simulink model "ScriptDemo"  (R2022b)
settings: configuration reference "TmVcThermal_Configuration_sub" (kept outside this file)
undefined symbols (not defined in the file): aaaa, bbbb, cTmComprCtrl_D_u8HvacFlowTable_db, cTmComprCtrl_D_u8HvacFlowTable_sw, cTmComprCtrl_n_i16ChillCmpIMax, cTmComprCtrl_n_i16ChillCmpIMin, cTmComprCtrl_n_i16ChillCmpIMin666, cTmComprCtrl_n_i16ChillCmpPMax, cTmComprCtrl_n_i16ChillCmpPMin, cTmComprCtrl_n_i16CmpChillCoolRpmKiMax, cTmComprCtrl_n_i16CmpChillCoolRpmKiMin, cTmComprCtrl_n_i16CmpChillCoolRpmKpMax, cTmComprCtrl_n_i16CmpChillCoolRpmKpMin, cTmComprCtrl_n_i16CmpCoolRpmKiMax, cTmComprCtrl_n_i16CmpCoolRpmKiMin, cTmComprCtrl_n_i16CmpCoolRpmKpMax, cTmComprCtrl_n_i16CmpCoolRpmKpMin, cTmComprCtrl_n_i16SM4CmpHeatKiMax, cTmComprCtrl_n_i16SM4CmpHeatKiMin, cTmComprCtrl_n_i16SM4CmpHeatKpMax, cTmComprCtrl_n_i16SM4CmpHeatKpMin, cTmComprCtrl_n_i16SM5CmpHeatKiMax, cTmComprCtrl_n_i16SM5CmpHeatKiMin, cTmComprCtrl_n_i16SM5CmpHeatKpMax, cTmComprCtrl_n_i16SM5CmpHeatKpMin, cTmComprCtrl_n_i16SM6CmpHeatKiMax, cTmComprCtrl_n_i16SM6CmpHeatKiMin, cTmComprCtrl_n_i16SM6CmpHeatKpMax, cTmComprCtrl_n_i16SM6CmpHeatKpMin, cTmComprCtrl_n_u16CmpMaxSpdFanFltLimt, cTmComprCtrl_n_u16CmpMaxSpdLoSidePFltLimt, cTmComprCtrl_n_u16CmpMaxSpdSensorFltLimt, cTmComprCtrl_n_u16CompMinRpm, cTmComprCtrl_n_u16CompRpmIncThres, cTmComprCtrl_t_u16BattCooltFFPeriod, cTmComprCtrl_t_u16BattCooltPIPeriod, cTmComprCtrl_t_u16CmpCoolFFPeriod, cTmComprCtrl_t_u16CmpCoolPIPeriod, cTmComprCtrl_t_u16CoolCmpChillFFPeriod, cTmComprCtrl_t_u16CoolCmpChillPIPeriod, cTmComprCtrl_t_u16SM4CmpHeatFFPeriod, cTmComprCtrl_t_u16SM4CmpHeatPIPeriod, cTmComprCtrl_t_u16SM5CmpHeatFFPeriod, cTmComprCtrl_t_u16SM5CmpHeatPIPeriod, cTmComprCtrl_t_u16SM6CmpHeatFFPeriod, cTmComprCtrl_t_u16SM6CmpHeatPIPeriod, cTmComprCtrl_Te_EvapClearInteg, cTmComprCtrl_Te_i16HpReqTempSaturoffset, cTmComprCtrl_Te_i16SatLpReplaceDiff, cTmComprCtrl_Te_i16SM3BatDiffStartEvapDecOffset, cTmComprCtrl_Te_i16SM3EvapLo, cTmComprCtrl_Te_i16SM3TBatDiffEntEvapDecOffset, cTmComprCtrl_Te_i16SM3TBatDiffEntEvapDecOffsetQuit, cTmComprCtrl_Te_s32ErrCmpChillPIContinueCoolH, cTmComprCtrl_Te_s32ErrCmpChillPIContinueCoolL, cTmComprCtrl_Te_s32ErrCmpPIContinueChillH, cTmComprCtrl_Te_s32ErrCmpPIContinueChillL, cTmComprCtrl_Te_s32ErrCmpPIContinueCoolH, cTmComprCtrl_Te_s32ErrCmpPIContinueCoolL, cTmComprCtrl_Te_s32ErrCmpPIContinueHeatH ... (+398)
libraries: simulink x782, PCMULib x640, simulink_need_slupdate x4
(part 27 of 41)

== system ScriptDemo/Create/createMerge/Before/SM2SM22/ID26239_SM2Error/NegAndPosCheck 1 ==
  SetPoint : Inport
  Acture : Inport  Port=2
  Compare To Constant : simulink/Logic and Bit Operations/Compare To Constant  relop=>=  const=0  OutDataTypeStr=boolean
  Data Type Conversion : DataTypeConversion  SaturateOnIntegerOverflow=off  RndMeth=Floor
  Data Type Conversion1 : DataTypeConversion  SaturateOnIntegerOverflow=off  RndMeth=Floor
  Data Type Conversion2 : DataTypeConversion  SaturateOnIntegerOverflow=off  RndMeth=Floor
  Sum : Sum  Inputs=|-+  OutDataTypeStr=Inherit: Same as first input
  Dvt : Outport  VectorParamsAs1DForOutWhenUnconnected=off
  Dvt_PosFlag : Outport  Port=2  VectorParamsAs1DForOutWhenUnconnected=off
  wires:
  Data Type Conversion2/1 -> Dvt/1, Compare To Constant/1
  Data Type Conversion1/1 -> Sum/2
  Data Type Conversion/1 -> Sum/1
  Compare To Constant/1 -> Dvt_PosFlag/1
  Sum/1 -> Data Type Conversion2/1
  Acture/1 -> Data Type Conversion1/1
  SetPoint/1 -> Data Type Conversion/1

== system ScriptDemo/Create/createMerge/Before/SM2SM22/ID26267_SM2FF/Flow2RpmOsa ==
  md_u8Blw : Inport
  breakpoint1 : Inport  Port=2
  breakpoint2 : Inport  Port=3
  2-D Lookup Table5 : Lookup_n-D  BreakpointsForDimension1=FFBlw1_Y  BreakpointsForDimension2=FFBlw1_X  BreakpointsForDimension1DataTypeStr=Inherit: Inherit from 'Breakpoint data'  BreakpointsForDimension2DataTypeStr=Inherit: Inherit from 'Breakpoint data'  Table=FFBlw1  TableDataTypeStr=Inherit: Inherit from 'Table data'  ExtrapMethod=Clip  InternalRulePriority=Speed  OutDataTypeStr=Inherit: Inherit from 'Table data'  RndMeth=Simplest
      settings: InputPortMap=u0,u1
  2-D Lookup Table6 : Lookup_n-D  BreakpointsForDimension1=FFBlw3_Y  BreakpointsForDimension2=FFBlw3_X  BreakpointsForDimension1DataTypeStr=Inherit: Inherit from 'Breakpoint data'  BreakpointsForDimension2DataTypeStr=Inherit: Inherit from 'Breakpoint data'  Table=FFBlw3  TableDataTypeStr=Inherit: Inherit from 'Table data'  ExtrapMethod=Clip  InternalRulePriority=Speed  OutDataTypeStr=Inherit: Inherit from 'Table data'  RndMeth=Simplest
      settings: InputPortMap=u0,u1
  2-D Lookup Table7 : Lookup_n-D  BreakpointsForDimension1=FFBlw5_Y  BreakpointsForDimension2=FFBlw5_X  BreakpointsForDimension1DataTypeStr=Inherit: Inherit from 'Breakpoint data'  BreakpointsForDimension2DataTypeStr=Inherit: Inherit from 'Breakpoint data'  Table=FFBlw5  TableDataTypeStr=Inherit: Inherit from 'Table data'  ExtrapMethod=Clip  InternalRulePriority=Speed  OutDataTypeStr=Inherit: Inherit from 'Table data'  RndMeth=Simplest
      settings: InputPortMap=u0,u1
  2-D Lookup Table8 : Lookup_n-D  BreakpointsForDimension1=FFBlw7_Y  BreakpointsForDimension2=FFBlw7_X  BreakpointsForDimension1DataTypeStr=Inherit: Inherit from 'Breakpoint data'  BreakpointsForDimension2DataTypeStr=Inherit: Inherit from 'Breakpoint data'  Table=FFBlw7  TableDataTypeStr=Inherit: Inherit from 'Table data'  ExtrapMethod=Clip  InternalRulePriority=Speed  OutDataTypeStr=Inherit: Inherit from 'Table data'  RndMeth=Simplest
      settings: InputPortMap=u0,u1
  2-D Lookup Table9 : Lookup_n-D  BreakpointsForDimension1=FFBlw9_Y  BreakpointsForDimension2=FFBlw9_X  BreakpointsForDimension1DataTypeStr=Inherit: Inherit from 'Breakpoint data'  BreakpointsForDimension2DataTypeStr=Inherit: Inherit from 'Breakpoint data'  Table=FFBlw9  TableDataTypeStr=Inherit: Inherit from 'Table data'  ExtrapMethod=Clip  InternalRulePriority=Speed  OutDataTypeStr=Inherit: Inherit from 'Table data'  RndMeth=Simplest
      settings: InputPortMap=u0,u1
  Add{2..6} (5 alike) : Sum  Inputs=+-  OutDataTypeStr=int16
  Add7 : Sum  Inputs=+++++
  Constant{,1..4} (5 alike) : Constant  Value=0.1  OutDataTypeStr=single
  Constant5 : Constant  Value=10  OutDataTypeStr=int16
  Constant6 : Constant  Value=20  OutDataTypeStr=int16
  Constant7 : Constant  Value=30  OutDataTypeStr=int16
  Constant8 : Constant  Value=40  OutDataTypeStr=int16
  Constant9 : Constant  Value=50  OutDataTypeStr=int16
  Data Type Conversion : DataTypeConversion  OutDataTypeStr=uint16  SaturateOnIntegerOverflow=off  RndMeth=Floor
  Data Type Conversion1 : DataTypeConversion  OutDataTypeStr=int16  SaturateOnIntegerOverflow=off  RndMeth=Floor
  Product{,1..9} (10 alike) : Product  OutDataTypeStr=single
  Subsystem1 : Subsystem
  Subsystem2 : Subsystem
  Subsystem3 : Subsystem
  Subsystem4 : Subsystem
  Subsystem5 : Subsystem
  XCP : Subsystem
  Flow2Rpm : Outport
  wires:
  Subsystem1/1(Out1) -> Product/2
  Product2/1 -> Product7/2
  [breakpoint2] -> 2-D Lookup Table5/2
  Product4/1 -> Product9/2
  Product9/1 -> Add7/5
  [breakpoint1] -> 2-D Lookup Table7/1
  Constant9/1 -> Add6/1
  [breakpoint1] -> 2-D Lookup Table9/1
  [breakpoint1] -> 2-D Lookup Table5/1
  [breakpoint1] -> 2-D Lookup Table6/1
  Product5/1 -> Add7/1
  2-D Lookup Table7/1 -> Product2/1
  Data Type Conversion1/1 -> Add4/2, Add6/2, Add5/2, Add3/2, Add2/2
  [breakpoint2] -> 2-D Lookup Table8/2
  Product/1 -> Product5/2
  Subsystem5/1(Out1) -> Product4/2
  [breakpoint2] -> 2-D Lookup Table7/2
  Subsystem2/1(Out1) -> Product1/2
  Constant8/1 -> Add5/1
  Product8/1 -> Add7/4
  Constant7/1 -> Add4/1
  Add4/1 -> Subsystem3/1(In1)
  Subsystem3/1(Out1) -> Product2/2
  Subsystem4/1(Out1) -> Product3/2
  Product1/1 -> Product6/2
  Add2/1 -> Subsystem1/1(In1)
  [breakpoint1] -> 2-D Lookup Table8/1
  [breakpoint2] -> 2-D Lookup Table6/2
  2-D Lookup Table5/1 -> Product/1
  Constant5/1 -> Add2/1
  2-D Lookup Table8/1 -> Product3/1
  Constant6/1 -> Add3/1
  Add6/1 -> Subsystem5/1(In1)
  Add5/1 -> Subsystem4/1(In1)
  Product3/1 -> Product8/2
  [breakpoint2] -> 2-D Lookup Table9/2
  Add3/1 -> Subsystem2/1(In1)
  Add7/1 -> Data Type Conversion/1
  2-D Lookup Table6/1 -> Product1/1
  Product7/1 -> Add7/3
  2-D Lookup Table9/1 -> Product4/1
  Product6/1 -> Add7/2
  breakpoint1/1 -> [breakpoint1]
  breakpoint2/1 -> [breakpoint2]
  XCP/1(Out1) -> Data Type Conversion1/1
  Constant/1 -> Product5/1
  Constant1/1 -> Product6/1
  Constant2/1 -> Product7/1
  Constant3/1 -> Product8/1
  Constant4/1 -> Product9/1
  md_u8Blw/1 -> XCP/1(md_u8Blw)
  Data Type Conversion/1 -> Flow2Rpm/1

== system ScriptDemo/Create/createMerge/Before/SM2SM22/ID26267_SM2FF/Flow2RpmOsa1 ==
  md_u8Blw : Inport
  breakpoint1 : Inport  Port=2
  breakpoint2 : Inport  Port=3
  2-D Lookup Table5 : Lookup_n-D  BreakpointsForDimension1=FFBlw1_Y  BreakpointsForDimension2=FFBlw1_X  BreakpointsForDimension1DataTypeStr=Inherit: Inherit from 'Breakpoint data'  BreakpointsForDimension2DataTypeStr=Inherit: Inherit from 'Breakpoint data'  Table=FFBlw1  TableDataTypeStr=Inherit: Inherit from 'Table data'  ExtrapMethod=Clip  InternalRulePriority=Speed  OutDataTypeStr=Inherit: Inherit from 'Table data'  RndMeth=Simplest
      settings: InputPortMap=u0,u1
  2-D Lookup Table6 : Lookup_n-D  BreakpointsForDimension1=FFBlw3_Y  BreakpointsForDimension2=FFBlw3_X  BreakpointsForDimension1DataTypeStr=Inherit: Inherit from 'Breakpoint data'  BreakpointsForDimension2DataTypeStr=Inherit: Inherit from 'Breakpoint data'  Table=FFBlw3  TableDataTypeStr=Inherit: Inherit from 'Table data'  ExtrapMethod=Clip  InternalRulePriority=Speed  OutDataTypeStr=Inherit: Inherit from 'Table data'  RndMeth=Simplest
      settings: InputPortMap=u0,u1
  2-D Lookup Table7 : Lookup_n-D  BreakpointsForDimension1=FFBlw5_Y  BreakpointsForDimension2=FFBlw5_X  BreakpointsForDimension1DataTypeStr=Inherit: Inherit from 'Breakpoint data'  BreakpointsForDimension2DataTypeStr=Inherit: Inherit from 'Breakpoint data'  Table=FFBlw5  TableDataTypeStr=Inherit: Inherit from 'Table data'  ExtrapMethod=Clip  InternalRulePriority=Speed  OutDataTypeStr=Inherit: Inherit from 'Table data'  RndMeth=Simplest
      settings: InputPortMap=u0,u1
  2-D Lookup Table8 : Lookup_n-D  BreakpointsForDimension1=FFBlw7_Y  BreakpointsForDimension2=FFBlw7_X  BreakpointsForDimension1DataTypeStr=Inherit: Inherit from 'Breakpoint data'  BreakpointsForDimension2DataTypeStr=Inherit: Inherit from 'Breakpoint data'  Table=FFBlw7  TableDataTypeStr=Inherit: Inherit from 'Table data'  ExtrapMethod=Clip  InternalRulePriority=Speed  OutDataTypeStr=Inherit: Inherit from 'Table data'  RndMeth=Simplest
      settings: InputPortMap=u0,u1
  2-D Lookup Table9 : Lookup_n-D  BreakpointsForDimension1=FFBlw9_Y  BreakpointsForDimension2=FFBlw9_X  BreakpointsForDimension1DataTypeStr=Inherit: Inherit from 'Breakpoint data'  BreakpointsForDimension2DataTypeStr=Inherit: Inherit from 'Breakpoint data'  Table=FFBlw9  TableDataTypeStr=Inherit: Inherit from 'Table data'  ExtrapMethod=Clip  InternalRulePriority=Speed  OutDataTypeStr=Inherit: Inherit from 'Table data'  RndMeth=Simplest
      settings: InputPortMap=u0,u1
  Add{2..6} (5 alike) : Sum  Inputs=+-  OutDataTypeStr=int16
  Add7 : Sum  Inputs=+++++
  Constant{,1..4} (5 alike) : Constant  Value=0.1  OutDataTypeStr=single
  Constant5 : Constant  Value=10  OutDataTypeStr=int16
  Constant6 : Constant  Value=20  OutDataTypeStr=int16
  Constant7 : Constant  Value=30  OutDataTypeStr=int16
  Constant8 : Constant  Value=40  OutDataTypeStr=int16
  Constant9 : Constant  Value=50  OutDataTypeStr=int16
  Data Type Conversion : DataTypeConversion  OutDataTypeStr=uint16  SaturateOnIntegerOverflow=off  RndMeth=Floor
  Data Type Conversion1 : DataTypeConversion  OutDataTypeStr=int16  SaturateOnIntegerOverflow=off  RndMeth=Floor
  Product{,1..9} (10 alike) : Product  OutDataTypeStr=single
  Subsystem1 : Subsystem
  Subsystem2 : Subsystem
  Subsystem3 : Subsystem
  Subsystem4 : Subsystem
  Subsystem5 : Subsystem
  XCP : Subsystem
  Flow2Rpm : Outport
  wires:
  Subsystem1/1(Out1) -> Product/2
  Product2/1 -> Product7/2
  [breakpoint2] -> 2-D Lookup Table5/2
  Product4/1 -> Product9/2
  Product9/1 -> Add7/5
  [breakpoint1] -> 2-D Lookup Table7/1
  Constant9/1 -> Add6/1
  [breakpoint1] -> 2-D Lookup Table9/1
  [breakpoint1] -> 2-D Lookup Table5/1
  [breakpoint1] -> 2-D Lookup Table6/1
  Product5/1 -> Add7/1
  2-D Lookup Table7/1 -> Product2/1
  Data Type Conversion1/1 -> Add4/2, Add6/2, Add5/2, Add3/2, Add2/2
  [breakpoint2] -> 2-D Lookup Table8/2
  Product/1 -> Product5/2
  Subsystem5/1(Out1) -> Product4/2
  [breakpoint2] -> 2-D Lookup Table7/2
  Subsystem2/1(Out1) -> Product1/2
  Constant8/1 -> Add5/1
  Product8/1 -> Add7/4
  Constant7/1 -> Add4/1
  Add4/1 -> Subsystem3/1(In1)
  Subsystem3/1(Out1) -> Product2/2
  Subsystem4/1(Out1) -> Product3/2
  Product1/1 -> Product6/2
  Add2/1 -> Subsystem1/1(In1)
  [breakpoint1] -> 2-D Lookup Table8/1
  [breakpoint2] -> 2-D Lookup Table6/2
  2-D Lookup Table5/1 -> Product/1
  Constant5/1 -> Add2/1
  2-D Lookup Table8/1 -> Product3/1
  Constant6/1 -> Add3/1
  Add6/1 -> Subsystem5/1(In1)
  Add5/1 -> Subsystem4/1(In1)
  Product3/1 -> Product8/2
  [breakpoint2] -> 2-D Lookup Table9/2
  Add3/1 -> Subsystem2/1(In1)
  Add7/1 -> Data Type Conversion/1
  2-D Lookup Table6/1 -> Product1/1
  Product7/1 -> Add7/3
  2-D Lookup Table9/1 -> Product4/1
  Product6/1 -> Add7/2
  breakpoint1/1 -> [breakpoint1]
  breakpoint2/1 -> [breakpoint2]
  XCP/1(Out1) -> Data Type Conversion1/1
  Constant/1 -> Product5/1
  Constant1/1 -> Product6/1
  Constant2/1 -> Product7/1
  Constant3/1 -> Product8/1
  Constant4/1 -> Product9/1
  md_u8Blw/1 -> XCP/1(md_u8Blw)
  Data Type Conversion/1 -> Flow2Rpm/1

== system ScriptDemo/Create/createMerge/Before/SM2SM22/ID26267_SM2FF/Flow2RpmRec ==
  md_u8Blw : Inport
  breakpoint1 : Inport  Port=2
  breakpoint2 : Inport  Port=3
  2-D Lookup Table5 : Lookup_n-D  BreakpointsForDimension1=FFBlw1_Y  BreakpointsForDimension2=FFBlw1_X  BreakpointsForDimension1DataTypeStr=Inherit: Inherit from 'Breakpoint data'  BreakpointsForDimension2DataTypeStr=Inherit: Inherit from 'Breakpoint data'  Table=FFBlw1  TableDataTypeStr=Inherit: Inherit from 'Table data'  ExtrapMethod=Clip  InternalRulePriority=Speed  OutDataTypeStr=Inherit: Inherit from 'Table data'  RndMeth=Simplest
      settings: InputPortMap=u0,u1
  2-D Lookup Table6 : Lookup_n-D  BreakpointsForDimension1=FFBlw3_Y  BreakpointsForDimension2=FFBlw3_X  BreakpointsForDimension1DataTypeStr=Inherit: Inherit from 'Breakpoint data'  BreakpointsForDimension2DataTypeStr=Inherit: Inherit from 'Breakpoint data'  Table=FFBlw3  TableDataTypeStr=Inherit: Inherit from 'Table data'  ExtrapMethod=Clip  InternalRulePriority=Speed  OutDataTypeStr=Inherit: Inherit from 'Table data'  RndMeth=Simplest
      settings: InputPortMap=u0,u1
  2-D Lookup Table7 : Lookup_n-D  BreakpointsForDimension1=FFBlw5_Y  BreakpointsForDimension2=FFBlw5_X  BreakpointsForDimension1DataTypeStr=Inherit: Inherit from 'Breakpoint data'  BreakpointsForDimension2DataTypeStr=Inherit: Inherit from 'Breakpoint data'  Table=FFBlw5  TableDataTypeStr=Inherit: Inherit from 'Table data'  ExtrapMethod=Clip  InternalRulePriority=Speed  OutDataTypeStr=Inherit: Inherit from 'Table data'  RndMeth=Simplest
      settings: InputPortMap=u0,u1
  2-D Lookup Table8 : Lookup_n-D  BreakpointsForDimension1=FFBlw7_Y  BreakpointsForDimension2=FFBlw7_X  BreakpointsForDimension1DataTypeStr=Inherit: Inherit from 'Breakpoint data'  BreakpointsForDimension2DataTypeStr=Inherit: Inherit from 'Breakpoint data'  Table=FFBlw7  TableDataTypeStr=Inherit: Inherit from 'Table data'  ExtrapMethod=Clip  InternalRulePriority=Speed  OutDataTypeStr=Inherit: Inherit from 'Table data'  RndMeth=Simplest
      settings: InputPortMap=u0,u1
  2-D Lookup Table9 : Lookup_n-D  BreakpointsForDimension1=FFBlw9_Y  BreakpointsForDimension2=FFBlw9_X  BreakpointsForDimension1DataTypeStr=Inherit: Inherit from 'Breakpoint data'  BreakpointsForDimension2DataTypeStr=Inherit: Inherit from 'Breakpoint data'  Table=FFBlw9  TableDataTypeStr=Inherit: Inherit from 'Table data'  ExtrapMethod=Clip  InternalRulePriority=Speed  OutDataTypeStr=Inherit: Inherit from 'Table data'  RndMeth=Simplest
      settings: InputPortMap=u0,u1
  Add{2..6} (5 alike) : Sum  Inputs=+-  OutDataTypeStr=int16
  Add7 : Sum  Inputs=+++++
  Constant{,1..4} (5 alike) : Constant  Value=0.1  OutDataTypeStr=single
  Constant5 : Constant  Value=10  OutDataTypeStr=int16
  Constant6 : Constant  Value=20  OutDataTypeStr=int16
  Constant7 : Constant  Value=30  OutDataTypeStr=int16
  Constant8 : Constant  Value=40  OutDataTypeStr=int16
  Constant9 : Constant  Value=50  OutDataTypeStr=int16
  Data Type Conversion : DataTypeConversion  OutDataTypeStr=uint16  SaturateOnIntegerOverflow=off  RndMeth=Floor
  Data Type Conversion1 : DataTypeConversion  OutDataTypeStr=int16  SaturateOnIntegerOverflow=off  RndMeth=Floor
  Product{,1..9} (10 alike) : Product  OutDataTypeStr=single
  Subsystem1 : Subsystem
  Subsystem2 : Subsystem
  Subsystem3 : Subsystem
  Subsystem4 : Subsystem
  Subsystem5 : Subsystem
  XCP : Subsystem
  Flow2Rpm : Outport
  wires:
  Subsystem1/1(Out1) -> Product/2
  Product2/1 -> Product7/2
  [breakpoint2] -> 2-D Lookup Table5/2
  Product4/1 -> Product9/2
  Product9/1 -> Add7/5
  [breakpoint1] -> 2-D Lookup Table7/1
  Constant9/1 -> Add6/1
  [breakpoint1] -> 2-D Lookup Table9/1
  [breakpoint1] -> 2-D Lookup Table5/1
  [breakpoint1] -> 2-D Lookup Table6/1
  Product5/1 -> Add7/1
  2-D Lookup Table7/1 -> Product2/1
  Data Type Conversion1/1 -> Add4/2, Add6/2, Add5/2, Add3/2, Add2/2
  [breakpoint2] -> 2-D Lookup Table8/2
  Product/1 -> Product5/2
  Subsystem5/1(Out1) -> Product4/2
  [breakpoint2] -> 2-D Lookup Table7/2
  Subsystem2/1(Out1) -> Product1/2
  Constant8/1 -> Add5/1
  Product8/1 -> Add7/4
  Constant7/1 -> Add4/1
  Add4/1 -> Subsystem3/1(In1)
  Subsystem3/1(Out1) -> Product2/2
  Subsystem4/1(Out1) -> Product3/2
  Product1/1 -> Product6/2
  Add2/1 -> Subsystem1/1(In1)
  [breakpoint1] -> 2-D Lookup Table8/1
  [breakpoint2] -> 2-D Lookup Table6/2
  2-D Lookup Table5/1 -> Product/1
  Constant5/1 -> Add2/1
  2-D Lookup Table8/1 -> Product3/1
  Constant6/1 -> Add3/1
  Add6/1 -> Subsystem5/1(In1)
  Add5/1 -> Subsystem4/1(In1)
  Product3/1 -> Product8/2
  [breakpoint2] -> 2-D Lookup Table9/2
  Add3/1 -> Subsystem2/1(In1)
  Add7/1 -> Data Type Conversion/1
  2-D Lookup Table6/1 -> Product1/1
  Product7/1 -> Add7/3
  2-D Lookup Table9/1 -> Product4/1
  Product6/1 -> Add7/2
  breakpoint1/1 -> [breakpoint1]
  breakpoint2/1 -> [breakpoint2]
  XCP/1(Out1) -> Data Type Conversion1/1
  Constant/1 -> Product5/1
  Constant1/1 -> Product6/1
  Constant2/1 -> Product7/1
  Constant3/1 -> Product8/1
  Constant4/1 -> Product9/1
  md_u8Blw/1 -> XCP/1(md_u8Blw)
  Data Type Conversion/1 -> Flow2Rpm/1

== system ScriptDemo/Create/createMerge/Before/SM2SM22/ID26267_SM2FF/Flow2RpmRec1 ==
  md_u8Blw : Inport
  breakpoint1 : Inport  Port=2
  breakpoint2 : Inport  Port=3
  2-D Lookup Table5 : Lookup_n-D  BreakpointsForDimension1=FFBlw1_Y  BreakpointsForDimension2=FFBlw1_X  BreakpointsForDimension1DataTypeStr=Inherit: Inherit from 'Breakpoint data'  BreakpointsForDimension2DataTypeStr=Inherit: Inherit from 'Breakpoint data'  Table=FFBlw1  TableDataTypeStr=Inherit: Inherit from 'Table data'  ExtrapMethod=Clip  InternalRulePriority=Speed  OutDataTypeStr=Inherit: Inherit from 'Table data'  RndMeth=Simplest
      settings: InputPortMap=u0,u1
  2-D Lookup Table6 : Lookup_n-D  BreakpointsForDimension1=FFBlw3_Y  BreakpointsForDimension2=FFBlw3_X  BreakpointsForDimension1DataTypeStr=Inherit: Inherit from 'Breakpoint data'  BreakpointsForDimension2DataTypeStr=Inherit: Inherit from 'Breakpoint data'  Table=FFBlw3  TableDataTypeStr=Inherit: Inherit from 'Table data'  ExtrapMethod=Clip  InternalRulePriority=Speed  OutDataTypeStr=Inherit: Inherit from 'Table data'  RndMeth=Simplest
      settings: InputPortMap=u0,u1
  2-D Lookup Table7 : Lookup_n-D  BreakpointsForDimension1=FFBlw5_Y  BreakpointsForDimension2=FFBlw5_X  BreakpointsForDimension1DataTypeStr=Inherit: Inherit from 'Breakpoint data'  BreakpointsForDimension2DataTypeStr=Inherit: Inherit from 'Breakpoint data'  Table=FFBlw5  TableDataTypeStr=Inherit: Inherit from 'Table data'  ExtrapMethod=Clip  InternalRulePriority=Speed  OutDataTypeStr=Inherit: Inherit from 'Table data'  RndMeth=Simplest
      settings: InputPortMap=u0,u1
  2-D Lookup Table8 : Lookup_n-D  BreakpointsForDimension1=FFBlw7_Y  BreakpointsForDimension2=FFBlw7_X  BreakpointsForDimension1DataTypeStr=Inherit: Inherit from 'Breakpoint data'  BreakpointsForDimension2DataTypeStr=Inherit: Inherit from 'Breakpoint data'  Table=FFBlw7  TableDataTypeStr=Inherit: Inherit from 'Table data'  ExtrapMethod=Clip  InternalRulePriority=Speed  OutDataTypeStr=Inherit: Inherit from 'Table data'  RndMeth=Simplest
      settings: InputPortMap=u0,u1
  2-D Lookup Table9 : Lookup_n-D  BreakpointsForDimension1=FFBlw9_Y  BreakpointsForDimension2=FFBlw9_X  BreakpointsForDimension1DataTypeStr=Inherit: Inherit from 'Breakpoint data'  BreakpointsForDimension2DataTypeStr=Inherit: Inherit from 'Breakpoint data'  Table=FFBlw9  TableDataTypeStr=Inherit: Inherit from 'Table data'  ExtrapMethod=Clip  InternalRulePriority=Speed  OutDataTypeStr=Inherit: Inherit from 'Table data'  RndMeth=Simplest
      settings: InputPortMap=u0,u1
  Add{2..6} (5 alike) : Sum  Inputs=+-  OutDataTypeStr=int16
  Add7 : Sum  Inputs=+++++
  Constant{,1..4} (5 alike) : Constant  Value=0.1  OutDataTypeStr=single
  Constant5 : Constant  Value=10  OutDataTypeStr=int16
  Constant6 : Constant  Value=20  OutDataTypeStr=int16
  Constant7 : Constant  Value=30  OutDataTypeStr=int16
  Constant8 : Constant  Value=40  OutDataTypeStr=int16
  Constant9 : Constant  Value=50  OutDataTypeStr=int16
  Data Type Conversion : DataTypeConversion  OutDataTypeStr=uint16  SaturateOnIntegerOverflow=off  RndMeth=Floor
  Data Type Conversion1 : DataTypeConversion  OutDataTypeStr=int16  SaturateOnIntegerOverflow=off  RndMeth=Floor
  Product{,1..9} (10 alike) : Product  OutDataTypeStr=single
  Subsystem1 : Subsystem
  Subsystem2 : Subsystem
  Subsystem3 : Subsystem
  Subsystem4 : Subsystem
  Subsystem5 : Subsystem
  XCP : Subsystem
  Flow2Rpm : Outport
  wires:
  Subsystem1/1(Out1) -> Product/2
  Product2/1 -> Product7/2
  [breakpoint2] -> 2-D Lookup Table5/2
  Product4/1 -> Product9/2
  Product9/1 -> Add7/5
  [breakpoint1] -> 2-D Lookup Table7/1
  Constant9/1 -> Add6/1
  [breakpoint1] -> 2-D Lookup Table9/1
  [breakpoint1] -> 2-D Lookup Table5/1
  [breakpoint1] -> 2-D Lookup Table6/1
  Product5/1 -> Add7/1
  2-D Lookup Table7/1 -> Product2/1
  Data Type Conversion1/1 -> Add4/2, Add6/2, Add5/2, Add3/2, Add2/2
  [breakpoint2] -> 2-D Lookup Table8/2
  Product/1 -> Product5/2
  Subsystem5/1(Out1) -> Product4/2
  [breakpoint2] -> 2-D Lookup Table7/2
  Subsystem2/1(Out1) -> Product1/2
  Constant8/1 -> Add5/1
  Product8/1 -> Add7/4
  Constant7/1 -> Add4/1
  Add4/1 -> Subsystem3/1(In1)
  Subsystem3/1(Out1) -> Product2/2
  Subsystem4/1(Out1) -> Product3/2
  Product1/1 -> Product6/2
  Add2/1 -> Subsystem1/1(In1)
  [breakpoint1] -> 2-D Lookup Table8/1
  [breakpoint2] -> 2-D Lookup Table6/2
  2-D Lookup Table5/1 -> Product/1
  Constant5/1 -> Add2/1
  2-D Lookup Table8/1 -> Product3/1
  Constant6/1 -> Add3/1
  Add6/1 -> Subsystem5/1(In1)
  Add5/1 -> Subsystem4/1(In1)
  Product3/1 -> Product8/2
  [breakpoint2] -> 2-D Lookup Table9/2
  Add3/1 -> Subsystem2/1(In1)
  Add7/1 -> Data Type Conversion/1
  2-D Lookup Table6/1 -> Product1/1
  Product7/1 -> Add7/3
  2-D Lookup Table9/1 -> Product4/1
  Product6/1 -> Add7/2
  breakpoint1/1 -> [breakpoint1]
  breakpoint2/1 -> [breakpoint2]
  XCP/1(Out1) -> Data Type Conversion1/1
  Constant/1 -> Product5/1
  Constant1/1 -> Product6/1
  Constant2/1 -> Product7/1
  Constant3/1 -> Product8/1
  Constant4/1 -> Product9/1
  md_u8Blw/1 -> XCP/1(md_u8Blw)
  Data Type Conversion/1 -> Flow2Rpm/1

== system ScriptDemo/Create/createMerge/Before/SM2SM22/SM2FFEnable/PeriodTrig ==
  Counter_Reset : Inport
  Add : Sum
  Add1 : Sum  Inputs=+-
  Constant : Constant  Value=CounterLim
  Constant1 : Constant  Value=cTmSwArch_t_s32SampleTime
      settings: AttributesFormatString=%<Value>
  Constant2 : Constant  Value=0  OutDataTypeStr=single
  Constant50 : Constant  Value=cTmSwArch_t_s32SampleTime
      settings: AttributesFormatString=%<Value>
  Logical Operator : Logic  Operator=OR  AllPortsSameDT=off  OutDataTypeStr=boolean
  Relational Operator : RelationalOperator  OutDataTypeStr=boolean  RndMeth=Simplest  InputSameDT=off
  Switch : Switch  Criteria=u2 ~= 0  SaturateOnIntegerOverflow=off  InputSameDT=off
  Switch1 : Switch  Criteria=u2 ~= 0  SaturateOnIntegerOverflow=off  InputSameDT=off
  Unit Delay : UnitDelay  SampleTime=-1  HasFrameUpgradeWarning=on
  Unit Delay1 : UnitDelay  SampleTime=-1  HasFrameUpgradeWarning=on
  Counter_Trig : Outport
  wires:
  Relational Operator/1 -> Unit Delay1/1, Counter_Trig/1
  [CounterLim] -> Relational Operator/2
  Add/1 -> Unit Delay/1, Relational Operator/1
  Unit Delay/1 -> Switch/3
  Switch/1 -> Add/2
  Constant1/1 -> Add/1
  Logical Operator/1 -> Switch/2
  Counter_Reset/1 -> Switch1/2, Logical Operator/1
  Unit Delay1/1 -> Logical Operator/2
  Constant2/1 -> Switch1/3
  Switch1/1 -> Switch/1
  Add1/1 -> Switch1/1
  Constant50/1 -> Add1/2
  Constant/1 -> [CounterLim]
  [CounterLim] -> Add1/1

== system ScriptDemo/Create/createMerge/Before/SM2SM22/SM2_Ki/Flow2Rpm ==
  md_u8Blw : Inport
  breakpoint1 : Inport  Port=2
  breakpoint2 : Inport  Port=3
  2-D Lookup Table5 : Lookup_n-D  BreakpointsForDimension1=FFBlw1_Y  BreakpointsForDimension2=FFBlw1_X  BreakpointsForDimension1DataTypeStr=Inherit: Inherit from 'Breakpoint data'  BreakpointsForDimension2DataTypeStr=Inherit: Inherit from 'Breakpoint data'  Table=FFBlw1  TableDataTypeStr=Inherit: Inherit from 'Table data'  ExtrapMethod=Clip  InternalRulePriority=Speed  OutDataTypeStr=Inherit: Inherit from 'Table data'  RndMeth=Simplest
      settings: InputPortMap=u0,u1
  2-D Lookup Table6 : Lookup_n-D  BreakpointsForDimension1=FFBlw3_Y  BreakpointsForDimension2=FFBlw3_X  BreakpointsForDimension1DataTypeStr=Inherit: Inherit from 'Breakpoint data'  BreakpointsForDimension2DataTypeStr=Inherit: Inherit from 'Breakpoint data'  Table=FFBlw3  TableDataTypeStr=Inherit: Inherit from 'Table data'  ExtrapMethod=Clip  InternalRulePriority=Speed  OutDataTypeStr=Inherit: Inherit from 'Table data'  RndMeth=Simplest
      settings: InputPortMap=u0,u1
  2-D Lookup Table7 : Lookup_n-D  BreakpointsForDimension1=FFBlw5_Y  BreakpointsForDimension2=FFBlw5_X  BreakpointsForDimension1DataTypeStr=Inherit: Inherit from 'Breakpoint data'  BreakpointsForDimension2DataTypeStr=Inherit: Inherit from 'Breakpoint data'  Table=FFBlw5  TableDataTypeStr=Inherit: Inherit from 'Table data'  ExtrapMethod=Clip  InternalRulePriority=Speed  OutDataTypeStr=Inherit: Inherit from 'Table data'  RndMeth=Simplest
      settings: InputPortMap=u0,u1
  2-D Lookup Table8 : Lookup_n-D  BreakpointsForDimension1=FFBlw7_Y  BreakpointsForDimension2=FFBlw7_X  BreakpointsForDimension1DataTypeStr=Inherit: Inherit from 'Breakpoint data'  BreakpointsForDimension2DataTypeStr=Inherit: Inherit from 'Breakpoint data'  Table=FFBlw7  TableDataTypeStr=Inherit: Inherit from 'Table data'  ExtrapMethod=Clip  InternalRulePriority=Speed  OutDataTypeStr=Inherit: Inherit from 'Table data'  RndMeth=Simplest
      settings: InputPortMap=u0,u1
  2-D Lookup Table9 : Lookup_n-D  BreakpointsForDimension1=FFBlw9_Y  BreakpointsForDimension2=FFBlw9_X  BreakpointsForDimension1DataTypeStr=Inherit: Inherit from 'Breakpoint data'  BreakpointsForDimension2DataTypeStr=Inherit: Inherit from 'Breakpoint data'  Table=FFBlw9  TableDataTypeStr=Inherit: Inherit from 'Table data'  ExtrapMethod=Clip  InternalRulePriority=Speed  OutDataTypeStr=Inherit: Inherit from 'Table data'  RndMeth=Simplest
      settings: InputPortMap=u0,u1
  Add{2..6} (5 alike) : Sum  Inputs=+-  OutDataTypeStr=int16
  Add7 : Sum  Inputs=+++++
  Constant{,1..4} (5 alike) : Constant  Value=0.1  OutDataTypeStr=single
  Constant5 : Constant  Value=10  OutDataTypeStr=int16
  Constant6 : Constant  Value=20  OutDataTypeStr=int16
  Constant7 : Constant  Value=30  OutDataTypeStr=int16
  Constant8 : Constant  Value=40  OutDataTypeStr=int16
  Constant9 : Constant  Value=50  OutDataTypeStr=int16
  Data Type Conversion : DataTypeConversion  OutDataTypeStr=uint16  SaturateOnIntegerOverflow=off  RndMeth=Floor
  Data Type Conversion1 : DataTypeConversion  OutDataTypeStr=int16  SaturateOnIntegerOverflow=off  RndMeth=Floor
  Product{,1..9} (10 alike) : Product  OutDataTypeStr=single
  Subsystem1 : Subsystem
  Subsystem2 : Subsystem
  Subsystem3 : Subsystem
  Subsystem4 : Subsystem
  Subsystem5 : Subsystem
  XCP : Subsystem
  Flow2Rpm : Outport
  wires:
  Subsystem1/1(Out1) -> Product/2
  Product2/1 -> Product7/2
  [breakpoint2] -> 2-D Lookup Table5/2
  Product4/1 -> Product9/2
  Product9/1 -> Add7/5
  [breakpoint1] -> 2-D Lookup Table7/1
  Constant9/1 -> Add6/1
  [breakpoint1] -> 2-D Lookup Table9/1
  [breakpoint1] -> 2-D Lookup Table5/1
  [breakpoint1] -> 2-D Lookup Table6/1
  Product5/1 -> Add7/1
  2-D Lookup Table7/1 -> Product2/1
  Data Type Conversion1/1 -> Add4/2, Add6/2, Add5/2, Add3/2, Add2/2
  [breakpoint2] -> 2-D Lookup Table8/2
  Product/1 -> Product5/2
  Subsystem5/1(Out1) -> Product4/2
  [breakpoint2] -> 2-D Lookup Table7/2
  Subsystem2/1(Out1) -> Product1/2
  Constant8/1 -> Add5/1
  Product8/1 -> Add7/4
  Constant7/1 -> Add4/1
  Add4/1 -> Subsystem3/1(In1)
  Subsystem3/1(Out1) -> Product2/2
  Subsystem4/1(Out1) -> Product3/2
  Product1/1 -> Product6/2
  Add2/1 -> Subsystem1/1(In1)
  [breakpoint1] -> 2-D Lookup Table8/1
  [breakpoint2] -> 2-D Lookup Table6/2
  2-D Lookup Table5/1 -> Product/1
  Constant5/1 -> Add2/1
  2-D Lookup Table8/1 -> Product3/1
  Constant6/1 -> Add3/1
  Add6/1 -> Subsystem5/1(In1)
  Add5/1 -> Subsystem4/1(In1)
  Product3/1 -> Product8/2
  [breakpoint2] -> 2-D Lookup Table9/2
  Add3/1 -> Subsystem2/1(In1)
  Add7/1 -> Data Type Conversion/1
  2-D Lookup Table6/1 -> Product1/1
  Product7/1 -> Add7/3
  2-D Lookup Table9/1 -> Product4/1
  Product6/1 -> Add7/2
  breakpoint1/1 -> [breakpoint1]
  breakpoint2/1 -> [breakpoint2]
  XCP/1(Out1) -> Data Type Conversion1/1
  Constant/1 -> Product5/1
  Constant1/1 -> Product6/1
  Constant2/1 -> Product7/1
  Constant3/1 -> Product8/1
  Constant4/1 -> Product9/1
  md_u8Blw/1 -> XCP/1(md_u8Blw)
  Data Type Conversion/1 -> Flow2Rpm/1

== system ScriptDemo/Create/createMerge/Before/SM2SM22/SM2_Ki/Flow2Rpm1 ==
  md_u8Blw : Inport
  breakpoint1 : Inport  Port=2
  breakpoint2 : Inport  Port=3
  2-D Lookup Table5 : Lookup_n-D  BreakpointsForDimension1=FFBlw1_Y  BreakpointsForDimension2=FFBlw1_X  BreakpointsForDimension1DataTypeStr=Inherit: Inherit from 'Breakpoint data'  BreakpointsForDimension2DataTypeStr=Inherit: Inherit from 'Breakpoint data'  Table=FFBlw1  TableDataTypeStr=Inherit: Inherit from 'Table data'  ExtrapMethod=Clip  InternalRulePriority=Speed  OutDataTypeStr=Inherit: Inherit from 'Table data'  RndMeth=Simplest
      settings: InputPortMap=u0,u1
  2-D Lookup Table6 : Lookup_n-D  BreakpointsForDimension1=FFBlw3_Y  BreakpointsForDimension2=FFBlw3_X  BreakpointsForDimension1DataTypeStr=Inherit: Inherit from 'Breakpoint data'  BreakpointsForDimension2DataTypeStr=Inherit: Inherit from 'Breakpoint data'  Table=FFBlw3  TableDataTypeStr=Inherit: Inherit from 'Table data'  ExtrapMethod=Clip  InternalRulePriority=Speed  OutDataTypeStr=Inherit: Inherit from 'Table data'  RndMeth=Simplest
      settings: InputPortMap=u0,u1
  2-D Lookup Table7 : Lookup_n-D  BreakpointsForDimension1=FFBlw5_Y  BreakpointsForDimension2=FFBlw5_X  BreakpointsForDimension1DataTypeStr=Inherit: Inherit from 'Breakpoint data'  BreakpointsForDimension2DataTypeStr=Inherit: Inherit from 'Breakpoint data'  Table=FFBlw5  TableDataTypeStr=Inherit: Inherit from 'Table data'  ExtrapMethod=Clip  InternalRulePriority=Speed  OutDataTypeStr=Inherit: Inherit from 'Table data'  RndMeth=Simplest
      settings: InputPortMap=u0,u1
  2-D Lookup Table8 : Lookup_n-D  BreakpointsForDimension1=FFBlw7_Y  BreakpointsForDimension2=FFBlw7_X  BreakpointsForDimension1DataTypeStr=Inherit: Inherit from 'Breakpoint data'  BreakpointsForDimension2DataTypeStr=Inherit: Inherit from 'Breakpoint data'  Table=FFBlw7  TableDataTypeStr=Inherit: Inherit from 'Table data'  ExtrapMethod=Clip  InternalRulePriority=Speed  OutDataTypeStr=Inherit: Inherit from 'Table data'  RndMeth=Simplest
      settings: InputPortMap=u0,u1
  2-D Lookup Table9 : Lookup_n-D  BreakpointsForDimension1=FFBlw9_Y  BreakpointsForDimension2=FFBlw9_X  BreakpointsForDimension1DataTypeStr=Inherit: Inherit from 'Breakpoint data'  BreakpointsForDimension2DataTypeStr=Inherit: Inherit from 'Breakpoint data'  Table=FFBlw9  TableDataTypeStr=Inherit: Inherit from 'Table data'  ExtrapMethod=Clip  InternalRulePriority=Speed  OutDataTypeStr=Inherit: Inherit from 'Table data'  RndMeth=Simplest
      settings: InputPortMap=u0,u1
  Add{2..6} (5 alike) : Sum  Inputs=+-  OutDataTypeStr=int16
  Add7 : Sum  Inputs=+++++
  Constant{,1..4} (5 alike) : Constant  Value=0.1  OutDataTypeStr=single
  Constant5 : Constant  Value=10  OutDataTypeStr=int16
  Constant6 : Constant  Value=20  OutDataTypeStr=int16
  Constant7 : Constant  Value=30  OutDataTypeStr=int16
  Constant8 : Constant  Value=40  OutDataTypeStr=int16
  Constant9 : Constant  Value=50  OutDataTypeStr=int16
  Data Type Conversion : DataTypeConversion  OutDataTypeStr=uint16  SaturateOnIntegerOverflow=off  RndMeth=Floor
  Data Type Conversion1 : DataTypeConversion  OutDataTypeStr=int16  SaturateOnIntegerOverflow=off  RndMeth=Floor
  Product{,1..9} (10 alike) : Product  OutDataTypeStr=single
  Subsystem1 : Subsystem
  Subsystem2 : Subsystem
  Subsystem3 : Subsystem
  Subsystem4 : Subsystem
  Subsystem5 : Subsystem
  XCP : Subsystem
  Flow2Rpm : Outport
  wires:
  Subsystem1/1(Out1) -> Product/2
  Product2/1 -> Product7/2
  [breakpoint2] -> 2-D Lookup Table5/2
  Product4/1 -> Product9/2
  Product9/1 -> Add7/5
  [breakpoint1] -> 2-D Lookup Table7/1
  Constant9/1 -> Add6/1
  [breakpoint1] -> 2-D Lookup Table9/1
  [breakpoint1] -> 2-D Lookup Table5/1
  [breakpoint1] -> 2-D Lookup Table6/1
  Product5/1 -> Add7/1
  2-D Lookup Table7/1 -> Product2/1
  Data Type Conversion1/1 -> Add4/2, Add6/2, Add5/2, Add3/2, Add2/2
  [breakpoint2] -> 2-D Lookup Table8/2
  Product/1 -> Product5/2
  Subsystem5/1(Out1) -> Product4/2
  [breakpoint2] -> 2-D Lookup Table7/2
  Subsystem2/1(Out1) -> Product1/2
  Constant8/1 -> Add5/1
  Product8/1 -> Add7/4
  Constant7/1 -> Add4/1
  Add4/1 -> Subsystem3/1(In1)
  Subsystem3/1(Out1) -> Product2/2
  Subsystem4/1(Out1) -> Product3/2
  Product1/1 -> Product6/2
  Add2/1 -> Subsystem1/1(In1)
  [breakpoint1] -> 2-D Lookup Table8/1
  [breakpoint2] -> 2-D Lookup Table6/2
  2-D Lookup Table5/1 -> Product/1
  Constant5/1 -> Add2/1
  2-D Lookup Table8/1 -> Product3/1
  Constant6/1 -> Add3/1
  Add6/1 -> Subsystem5/1(In1)
  Add5/1 -> Subsystem4/1(In1)
  Product3/1 -> Product8/2
  [breakpoint2] -> 2-D Lookup Table9/2
  Add3/1 -> Subsystem2/1(In1)
  Add7/1 -> Data Type Conversion/1
  2-D Lookup Table6/1 -> Product1/1
  Product7/1 -> Add7/3
  2-D Lookup Table9/1 -> Product4/1
  Product6/1 -> Add7/2
  breakpoint1/1 -> [breakpoint1]
  breakpoint2/1 -> [breakpoint2]
  XCP/1(Out1) -> Data Type Conversion1/1
  Constant/1 -> Product5/1
  Constant1/1 -> Product6/1
  Constant2/1 -> Product7/1
  Constant3/1 -> Product8/1
  Constant4/1 -> Product9/1
  md_u8Blw/1 -> XCP/1(md_u8Blw)
  Data Type Conversion/1 -> Flow2Rpm/1

== system ScriptDemo/Create/createMerge/Before/SM2SM22/SM2_Kp/Osa ==
  md_u8Blw : Inport
  breakpoint1 : Inport  Port=2
  breakpoint2 : Inport  Port=3
  2-D Lookup Table5 : Lookup_n-D  BreakpointsForDimension1=FFBlw1_Y  BreakpointsForDimension2=FFBlw1_X  BreakpointsForDimension1DataTypeStr=Inherit: Inherit from 'Breakpoint data'  BreakpointsForDimension2DataTypeStr=Inherit: Inherit from 'Breakpoint data'  Table=FFBlw1  TableDataTypeStr=Inherit: Inherit from 'Table data'  ExtrapMethod=Clip  InternalRulePriority=Speed  OutDataTypeStr=Inherit: Inherit from 'Table data'  RndMeth=Simplest
      settings: InputPortMap=u0,u1
  2-D Lookup Table6 : Lookup_n-D  BreakpointsForDimension1=FFBlw3_Y  BreakpointsForDimension2=FFBlw3_X  BreakpointsForDimension1DataTypeStr=Inherit: Inherit from 'Breakpoint data'  BreakpointsForDimension2DataTypeStr=Inherit: Inherit from 'Breakpoint data'  Table=FFBlw3  TableDataTypeStr=Inherit: Inherit from 'Table data'  ExtrapMethod=Clip  InternalRulePriority=Speed  OutDataTypeStr=Inherit: Inherit from 'Table data'  RndMeth=Simplest
      settings: InputPortMap=u0,u1
  2-D Lookup Table7 : Lookup_n-D  BreakpointsForDimension1=FFBlw5_Y  BreakpointsForDimension2=FFBlw5_X  BreakpointsForDimension1DataTypeStr=Inherit: Inherit from 'Breakpoint data'  BreakpointsForDimension2DataTypeStr=Inherit: Inherit from 'Breakpoint data'  Table=FFBlw5  TableDataTypeStr=Inherit: Inherit from 'Table data'  ExtrapMethod=Clip  InternalRulePriority=Speed  OutDataTypeStr=Inherit: Inherit from 'Table data'  RndMeth=Simplest
      settings: InputPortMap=u0,u1
  2-D Lookup Table8 : Lookup_n-D  BreakpointsForDimension1=FFBlw7_Y  BreakpointsForDimension2=FFBlw7_X  BreakpointsForDimension1DataTypeStr=Inherit: Inherit from 'Breakpoint data'  BreakpointsForDimension2DataTypeStr=Inherit: Inherit from 'Breakpoint data'  Table=FFBlw7  TableDataTypeStr=Inherit: Inherit from 'Table data'  ExtrapMethod=Clip  InternalRulePriority=Speed  OutDataTypeStr=Inherit: Inherit from 'Table data'  RndMeth=Simplest
      settings: InputPortMap=u0,u1
  2-D Lookup Table9 : Lookup_n-D  BreakpointsForDimension1=FFBlw9_Y  BreakpointsForDimension2=FFBlw9_X  BreakpointsForDimension1DataTypeStr=Inherit: Inherit from 'Breakpoint data'  BreakpointsForDimension2DataTypeStr=Inherit: Inherit from 'Breakpoint data'  Table=FFBlw9  TableDataTypeStr=Inherit: Inherit from 'Table data'  ExtrapMethod=Clip  InternalRulePriority=Speed  OutDataTypeStr=Inherit: Inherit from 'Table data'  RndMeth=Simplest
      settings: InputPortMap=u0,u1
  Add{2..6} (5 alike) : Sum  Inputs=+-  OutDataTypeStr=int16
  Add7 : Sum  Inputs=+++++
  Constant{,1..4} (5 alike) : Constant  Value=0.1  OutDataTypeStr=single
  Constant5 : Constant  Value=10  OutDataTypeStr=int16
  Constant6 : Constant  Value=20  OutDataTypeStr=int16
  Constant7 : Constant  Value=30  OutDataTypeStr=int16
  Constant8 : Constant  Value=40  OutDataTypeStr=int16
  Constant9 : Constant  Value=50  OutDataTypeStr=int16
  Data Type Conversion : DataTypeConversion  OutDataTypeStr=uint16  SaturateOnIntegerOverflow=off  RndMeth=Floor
  Data Type Conversion1 : DataTypeConversion  OutDataTypeStr=int16  SaturateOnIntegerOverflow=off  RndMeth=Floor
  Product{,1..9} (10 alike) : Product  OutDataTypeStr=single
  Subsystem1 : Subsystem
  Subsystem2 : Subsystem
  Subsystem3 : Subsystem
  Subsystem4 : Subsystem
  Subsystem5 : Subsystem
  XCP : Subsystem
  Flow2Rpm : Outport
  wires:
  Subsystem1/1(Out1) -> Product/2
  Product2/1 -> Product7/2
  [breakpoint2] -> 2-D Lookup Table5/2
  Product4/1 -> Product9/2
  Product9/1 -> Add7/5
  [breakpoint1] -> 2-D Lookup Table7/1
  Constant9/1 -> Add6/1
  [breakpoint1] -> 2-D Lookup Table9/1
  [breakpoint1] -> 2-D Lookup Table5/1
  [breakpoint1] -> 2-D Lookup Table6/1
  Product5/1 -> Add7/1
  2-D Lookup Table7/1 -> Product2/1
  Data Type Conversion1/1 -> Add4/2, Add6/2, Add5/2, Add3/2, Add2/2
  [breakpoint2] -> 2-D Lookup Table8/2
  Product/1 -> Product5/2
  Subsystem5/1(Out1) -> Product4/2
  [breakpoint2] -> 2-D Lookup Table7/2
  Subsystem2/1(Out1) -> Product1/2
  Constant8/1 -> Add5/1
  Product8/1 -> Add7/4
  Constant7/1 -> Add4/1
  Add4/1 -> Subsystem3/1(In1)
  Subsystem3/1(Out1) -> Product2/2
  Subsystem4/1(Out1) -> Product3/2
  Product1/1 -> Product6/2
  Add2/1 -> Subsystem1/1(In1)
  [breakpoint1] -> 2-D Lookup Table8/1
  [breakpoint2] -> 2-D Lookup Table6/2
  2-D Lookup Table5/1 -> Product/1
  Constant5/1 -> Add2/1
  2-D Lookup Table8/1 -> Product3/1
  Constant6/1 -> Add3/1
  Add6/1 -> Subsystem5/1(In1)
  Add5/1 -> Subsystem4/1(In1)
  Product3/1 -> Product8/2
  [breakpoint2] -> 2-D Lookup Table9/2
  Add3/1 -> Subsystem2/1(In1)
  Add7/1 -> Data Type Conversion/1
  2-D Lookup Table6/1 -> Product1/1
  Product7/1 -> Add7/3
  2-D Lookup Table9/1 -> Product4/1
  Product6/1 -> Add7/2
  breakpoint1/1 -> [breakpoint1]
  breakpoint2/1 -> [breakpoint2]
  XCP/1(Out1) -> Data Type Conversion1/1
  Constant/1 -> Product5/1
  Constant1/1 -> Product6/1
  Constant2/1 -> Product7/1
  Constant3/1 -> Product8/1
  Constant4/1 -> Product9/1
  md_u8Blw/1 -> XCP/1(md_u8Blw)
  Data Type Conversion/1 -> Flow2Rpm/1

== system ScriptDemo/Create/createMerge/Before/SM2SM22/SM2_Kp/Rec ==
  md_u8Blw : Inport
  breakpoint1 : Inport  Port=2
  breakpoint2 : Inport  Port=3
  2-D Lookup Table5 : Lookup_n-D  BreakpointsForDimension1=FFBlw1_Y  BreakpointsForDimension2=FFBlw1_X  BreakpointsForDimension1DataTypeStr=Inherit: Inherit from 'Breakpoint data'  BreakpointsForDimension2DataTypeStr=Inherit: Inherit from 'Breakpoint data'  Table=FFBlw1  TableDataTypeStr=Inherit: Inherit from 'Table data'  ExtrapMethod=Clip  InternalRulePriority=Speed  OutDataTypeStr=Inherit: Inherit from 'Table data'  RndMeth=Simplest
      settings: InputPortMap=u0,u1
  2-D Lookup Table6 : Lookup_n-D  BreakpointsForDimension1=FFBlw3_Y  BreakpointsForDimension2=FFBlw3_X  BreakpointsForDimension1DataTypeStr=Inherit: Inherit from 'Breakpoint data'  BreakpointsForDimension2DataTypeStr=Inherit: Inherit from 'Breakpoint data'  Table=FFBlw3  TableDataTypeStr=Inherit: Inherit from 'Table data'  ExtrapMethod=Clip  InternalRulePriority=Speed  OutDataTypeStr=Inherit: Inherit from 'Table data'  RndMeth=Simplest
      settings: InputPortMap=u0,u1
  2-D Lookup Table7 : Lookup_n-D  BreakpointsForDimension1=FFBlw5_Y  BreakpointsForDimension2=FFBlw5_X  BreakpointsForDimension1DataTypeStr=Inherit: Inherit from 'Breakpoint data'  BreakpointsForDimension2DataTypeStr=Inherit: Inherit from 'Breakpoint data'  Table=FFBlw5  TableDataTypeStr=Inherit: Inherit from 'Table data'  ExtrapMethod=Clip  InternalRulePriority=Speed  OutDataTypeStr=Inherit: Inherit from 'Table data'  RndMeth=Simplest
      settings: InputPortMap=u0,u1
  2-D Lookup Table8 : Lookup_n-D  BreakpointsForDimension1=FFBlw7_Y  BreakpointsForDimension2=FFBlw7_X  BreakpointsForDimension1DataTypeStr=Inherit: Inherit from 'Breakpoint data'  BreakpointsForDimension2DataTypeStr=Inherit: Inherit from 'Breakpoint data'  Table=FFBlw7  TableDataTypeStr=Inherit: Inherit from 'Table data'  ExtrapMethod=Clip  InternalRulePriority=Speed  OutDataTypeStr=Inherit: Inherit from 'Table data'  RndMeth=Simplest
      settings: InputPortMap=u0,u1
  2-D Lookup Table9 : Lookup_n-D  BreakpointsForDimension1=FFBlw9_Y  BreakpointsForDimension2=FFBlw9_X  BreakpointsForDimension1DataTypeStr=Inherit: Inherit from 'Breakpoint data'  BreakpointsForDimension2DataTypeStr=Inherit: Inherit from 'Breakpoint data'  Table=FFBlw9  TableDataTypeStr=Inherit: Inherit from 'Table data'  ExtrapMethod=Clip  InternalRulePriority=Speed  OutDataTypeStr=Inherit: Inherit from 'Table data'  RndMeth=Simplest
      settings: InputPortMap=u0,u1
  Add{2..6} (5 alike) : Sum  Inputs=+-  OutDataTypeStr=int16
  Add7 : Sum  Inputs=+++++
  Constant{,1..4} (5 alike) : Constant  Value=0.1  OutDataTypeStr=single
  Constant5 : Constant  Value=10  OutDataTypeStr=int16
  Constant6 : Constant  Value=20  OutDataTypeStr=int16
  Constant7 : Constant  Value=30  OutDataTypeStr=int16
  Constant8 : Constant  Value=40  OutDataTypeStr=int16
  Constant9 : Constant  Value=50  OutDataTypeStr=int16
  Data Type Conversion : DataTypeConversion  OutDataTypeStr=uint16  SaturateOnIntegerOverflow=off  RndMeth=Floor
  Data Type Conversion1 : DataTypeConversion  OutDataTypeStr=int16  SaturateOnIntegerOverflow=off  RndMeth=Floor
  Product{,1..9} (10 alike) : Product  OutDataTypeStr=single
  Subsystem1 : Subsystem
  Subsystem2 : Subsystem
  Subsystem3 : Subsystem
  Subsystem4 : Subsystem
  Subsystem5 : Subsystem
  XCP : Subsystem
  Flow2Rpm : Outport
  wires:
  Subsystem1/1(Out1) -> Product/2
  Product2/1 -> Product7/2
  [breakpoint2] -> 2-D Lookup Table5/2
  Product4/1 -> Product9/2
  Product9/1 -> Add7/5
  [breakpoint1] -> 2-D Lookup Table7/1
  Constant9/1 -> Add6/1
  [breakpoint1] -> 2-D Lookup Table9/1
  [breakpoint1] -> 2-D Lookup Table5/1
  [breakpoint1] -> 2-D Lookup Table6/1
  Product5/1 -> Add7/1
  2-D Lookup Table7/1 -> Product2/1
  Data Type Conversion1/1 -> Add4/2, Add6/2, Add5/2, Add3/2, Add2/2
  [breakpoint2] -> 2-D Lookup Table8/2
  Product/1 -> Product5/2
  Subsystem5/1(Out1) -> Product4/2
  [breakpoint2] -> 2-D Lookup Table7/2
  Subsystem2/1(Out1) -> Product1/2
  Constant8/1 -> Add5/1
  Product8/1 -> Add7/4
  Constant7/1 -> Add4/1
  Add4/1 -> Subsystem3/1(In1)
  Subsystem3/1(Out1) -> Product2/2
  Subsystem4/1(Out1) -> Product3/2
  Product1/1 -> Product6/2
  Add2/1 -> Subsystem1/1(In1)
  [breakpoint1] -> 2-D Lookup Table8/1
  [breakpoint2] -> 2-D Lookup Table6/2
  2-D Lookup Table5/1 -> Product/1
  Constant5/1 -> Add2/1
  2-D Lookup Table8/1 -> Product3/1
  Constant6/1 -> Add3/1
  Add6/1 -> Subsystem5/1(In1)
  Add5/1 -> Subsystem4/1(In1)
  Product3/1 -> Product8/2
  [breakpoint2] -> 2-D Lookup Table9/2
  Add3/1 -> Subsystem2/1(In1)
  Add7/1 -> Data Type Conversion/1
  2-D Lookup Table6/1 -> Product1/1
  Product7/1 -> Add7/3
  2-D Lookup Table9/1 -> Product4/1
  Product6/1 -> Add7/2
  breakpoint1/1 -> [breakpoint1]
  breakpoint2/1 -> [breakpoint2]
  XCP/1(Out1) -> Data Type Conversion1/1
  Constant/1 -> Product5/1
  Constant1/1 -> Product6/1
  Constant2/1 -> Product7/1
  Constant3/1 -> Product8/1
  Constant4/1 -> Product9/1
  md_u8Blw/1 -> XCP/1(md_u8Blw)
  Data Type Conversion/1 -> Flow2Rpm/1

== system ScriptDemo/Create/createMerge/Before/SM3SM23/ID26262_SM3FF/SM1FFEnable ==
  xTmComprCtrl_B_CompOnReqCompOn : Inport  OutDataTypeStr=boolean
  BevvFFPeriod : Subsystem  mask{CounterLim=cTmComprCtrl_t_u16BattCooltFFPeriod}
      mask DialogControl ParameterGroupVar Prompt: 参数
  Compare To Constant2 : simulink/Logic and Bit Operations/Compare To Constant  relop===  const=0  OutDataTypeStr=boolean
  Compare To Constant3 : simulink/Logic and Bit Operations/Compare To Constant  relop===  const=1  OutDataTypeStr=boolean
  Logical Operator3 : Logic  AllPortsSameDT=off  OutDataTypeStr=boolean
  Unit Delay : UnitDelay  SampleTime=-1  HasFrameUpgradeWarning=on
  SM1FFEnable_B_SM1FFEnable : Outport  OutDataTypeStr=boolean
  wires:
  Unit Delay/1 -> Compare To Constant2/1
  [xTmComprCtrl_B_CompOnReqCompOn] -> Compare To Constant3/1, Unit Delay/1
  Compare To Constant2/1 -> Logical Operator3/1
  Logical Operator3/1 -> BevvFFPeriod/1(Counter_Reset)
  BevvFFPeriod/1(Counter_Trig) -> SM1FFEnable_B_SM1FFEnable/1
  Compare To Constant3/1 -> Logical Operator3/2
  xTmComprCtrl_B_CompOnReqCompOn/1 -> [xTmComprCtrl_B_CompOnReqCompOn]

== system ScriptDemo/Create/createMerge/Before/SM3SM23/ID26262_SM3FF/SM2FFEnable ==
  xTmComprCtrl_B_CompOnReqCompOn : Inport  OutDataTypeStr=boolean
  Compare To Constant2 : simulink/Logic and Bit Operations/Compare To Constant  relop===  const=0  OutDataTypeStr=boolean
  Compare To Constant3 : simulink/Logic and Bit Operations/Compare To Constant  relop===  const=1  OutDataTypeStr=boolean
  Logical Operator3 : Logic  AllPortsSameDT=off  OutDataTypeStr=boolean
  PeriodTrig : Subsystem  mask{CounterLim=cTmComprCtrl_t_u16CoolCmpChillFFPeriod}
      mask DialogControl ParameterGroupVar Prompt: 参数
  Unit Delay : UnitDelay  SampleTime=-1  HasFrameUpgradeWarning=on
  SM2FFEnable_B_SM2FFEnable : Outport  OutDataTypeStr=boolean
  wires:
  Unit Delay/1 -> Compare To Constant2/1
  [xTmComprCtrl_B_CompOnReqCompOn] -> Compare To Constant3/1, Unit Delay/1
  Compare To Constant2/1 -> Logical Operator3/1
  Logical Operator3/1 -> PeriodTrig/1(Counter_Reset)
  Compare To Constant3/1 -> Logical Operator3/2
  xTmComprCtrl_B_CompOnReqCompOn/1 -> [xTmComprCtrl_B_CompOnReqCompOn]
  PeriodTrig/1(Counter_Trig) -> SM2FFEnable_B_SM2FFEnable/1
